simulink model "model"  (Simulink 8.0)
settings: Solver=ode45  StartTime=0.0  StopTime=30.0  MaxStep=0.1  MinStep=0.01  RelTol=1e-3
undefined symbols (not defined in the file or in its folder): a
settings Model: Creator=hake5  LastModifiedBy=hake5
settings OptimizationCC: SimCompilerOptimization=On

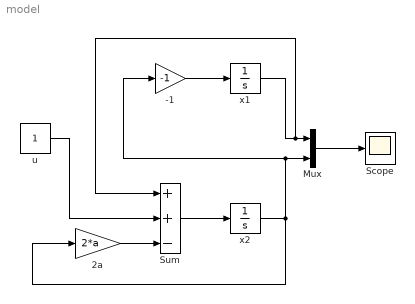
== system model ==
  -1 : Gain  Gain=-1
  2a : Gain  Gain=2*a
  Mux : Mux  Inputs=2
  Scope : Scope
  Sum : Sum  Inputs=++-
  u : Constant
  x1 : Integrator  InitialCondition=2
  x2 : Integrator  InitialCondition=1
  wires:
  Mux/1 -> Scope/1
  x1/1 -> Sum/1, Mux/1
  x2/1 -> 2a/1, Mux/2, -1/1
  Sum/1 -> x2/1
  -1/1 -> x1/1
  2a/1 -> Sum/3
  u/1 -> Sum/2
